simulink model "four_channel_bilateral_teleoperation_architecture"  (R2020b)
settings: Solver=VariableStepAuto  StartTime=0.0  StopTime=10.0  RelTol=1e-3
values from neighbouring files (symbols this model uses):
  A = 50    [four_channel_bilateral_teleoperation_architecture_params.m]    (also in four_channel_bilateral_teleoperation_kalman_params.m = 1; four_channel_bilateral_teleoperation_params.m = 1; kalman_test.m = [1 Ts Ts^2/2; 0 1 Ts; 0 0 1]; recursive_estimation.m = [1 Ts Ts^2/2; 0 1 Ts; 0 0 1])
  Be = 100    [four_channel_bilateral_teleoperation_architecture_params.m]    (also in four_channel_bilateral_teleoperation_kalman_params.m = 0; four_channel_bilateral_teleoperation_params.m = 0; scattering_based_bi_teleop_pf_kalman_params.m = 10; scattering_based_bi_teleop_pf_params.m = 10)
  Bh = 70    [four_channel_bilateral_teleoperation_architecture_params.m]    (also in four_channel_bilateral_teleoperation_kalman_params.m; four_channel_bilateral_teleoperation_params.m; scattering_based_bi_teleop_pf_kalman_params.m = 1.5; scattering_based_bi_teleop_pf_params.m = 1.5)
  Bm = 0.2    [four_channel_bilateral_teleoperation_architecture_params.m]    (also in four_channel_bilateral_teleoperation_kalman_params.m = 0.8; four_channel_bilateral_teleoperation_params.m = 0.8; scattering_based_bi_teleop_pf_kalman_params.m = 0; scattering_based_bi_teleop_pp_kalman_params.m = 15)
  Bs = 0.2    [four_channel_bilateral_teleoperation_architecture_params.m]    (also in four_channel_bilateral_teleoperation_kalman_params.m = 3.2; four_channel_bilateral_teleoperation_params.m = 3.2; scattering_based_bi_teleop_pf_kalman_params.m = 40; scattering_based_bi_teleop_pf_params.m = 3)
  Dh = 1.5    [four_channel_bilateral_teleoperation_architecture_params.m]    (also in four_channel_bilateral_teleoperation_kalman_params.m = 500; four_channel_bilateral_teleoperation_params.m = 100; scattering_based_bi_teleop_pf_kalman_params.m = 0; scattering_based_bi_teleop_pf_params.m = 17)
  Dm = 0    [four_channel_bilateral_teleoperation_architecture_params.m]    (also in four_channel_bilateral_teleoperation_kalman_params.m; four_channel_bilateral_teleoperation_params.m; scattering_based_bi_teleop_pf_kalman_params.m; scattering_based_bi_teleop_pf_params.m)
  Ds = 0    [four_channel_bilateral_teleoperation_architecture_params.m]    (also in four_channel_bilateral_teleoperation_kalman_params.m; four_channel_bilateral_teleoperation_params.m; scattering_based_bi_teleop_pf_kalman_params.m; scattering_based_bi_teleop_pf_params.m)
  Fc = 1    [four_channel_bilateral_teleoperation_architecture_params.m]    (also in four_channel_bilateral_teleoperation_kalman_params.m; four_channel_bilateral_teleoperation_params.m; kalman_test.m = 10; scattering_based_bi_teleop_pf_kalman_params.m = 0.1)
  Fip = 1    [four_channel_bilateral_teleoperation_architecture_params.m]    (also in four_channel_bilateral_teleoperation_kalman_params.m; four_channel_bilateral_teleoperation_params.m; scattering_based_bi_teleop_pf_kalman_params.m = 5; scattering_based_bi_teleop_pf_params.m)
  Je = 0    [four_channel_bilateral_teleoperation_architecture_params.m]    (also in four_channel_bilateral_teleoperation_kalman_params.m; four_channel_bilateral_teleoperation_params.m; scattering_based_bi_teleop_pf_kalman_params.m; scattering_based_bi_teleop_pf_params.m)
  Jh = 0.5    [four_channel_bilateral_teleoperation_architecture_params.m]    (also in four_channel_bilateral_teleoperation_kalman_params.m; four_channel_bilateral_teleoperation_params.m; scattering_based_bi_teleop_pf_kalman_params.m = 0; scattering_based_bi_teleop_pf_params.m = 0.05)
  Ke = 200    [four_channel_bilateral_teleoperation_architecture_params.m]    (also in four_channel_bilateral_teleoperation_kalman_params.m = 50; four_channel_bilateral_teleoperation_params.m; scattering_based_bi_teleop_pf_kalman_params.m; scattering_based_bi_teleop_pf_params.m)
  Kh = 2000    [four_channel_bilateral_teleoperation_architecture_params.m]    (also in four_channel_bilateral_teleoperation_kalman_params.m; four_channel_bilateral_teleoperation_params.m; scattering_based_bi_teleop_pf_kalman_params.m = 1; scattering_based_bi_teleop_pf_params.m = 0)
  Km = 30    [four_channel_bilateral_teleoperation_architecture_params.m]    (also in four_channel_bilateral_teleoperation_kalman_params.m = 1; four_channel_bilateral_teleoperation_params.m = 1; scattering_based_bi_teleop_pf_kalman_params.m = 0; scattering_based_bi_teleop_pp_kalman_params.m = 10)
  Ks = 30    [four_channel_bilateral_teleoperation_architecture_params.m]    (also in four_channel_bilateral_teleoperation_kalman_params.m = 4; four_channel_bilateral_teleoperation_params.m = 4; scattering_based_bi_teleop_pf_kalman_params.m = 50; scattering_based_bi_teleop_pf_params.m = 110)
  Mm = 0.5    [four_channel_bilateral_teleoperation_architecture_params.m]    (also in four_channel_bilateral_teleoperation_kalman_params.m; four_channel_bilateral_teleoperation_params.m; scattering_based_bi_teleop_pf_kalman_params.m; scattering_based_bi_teleop_pf_params.m)
  Ms = 2    [four_channel_bilateral_teleoperation_architecture_params.m]    (also in four_channel_bilateral_teleoperation_kalman_params.m; four_channel_bilateral_teleoperation_params.m; scattering_based_bi_teleop_pf_kalman_params.m; scattering_based_bi_teleop_pf_params.m)
  Ph = 0.2    [four_channel_bilateral_teleoperation_architecture_params.m]    (also in four_channel_bilateral_teleoperation_kalman_params.m = 2000; four_channel_bilateral_teleoperation_params.m = 20100; scattering_based_bi_teleop_pf_kalman_params.m = 5; scattering_based_bi_teleop_pf_params.m = 23)
  tau = 10000    [four_channel_bilateral_teleoperation_architecture_params.m]
settings Model: Creator=anuj  LastModifiedBy=filippo

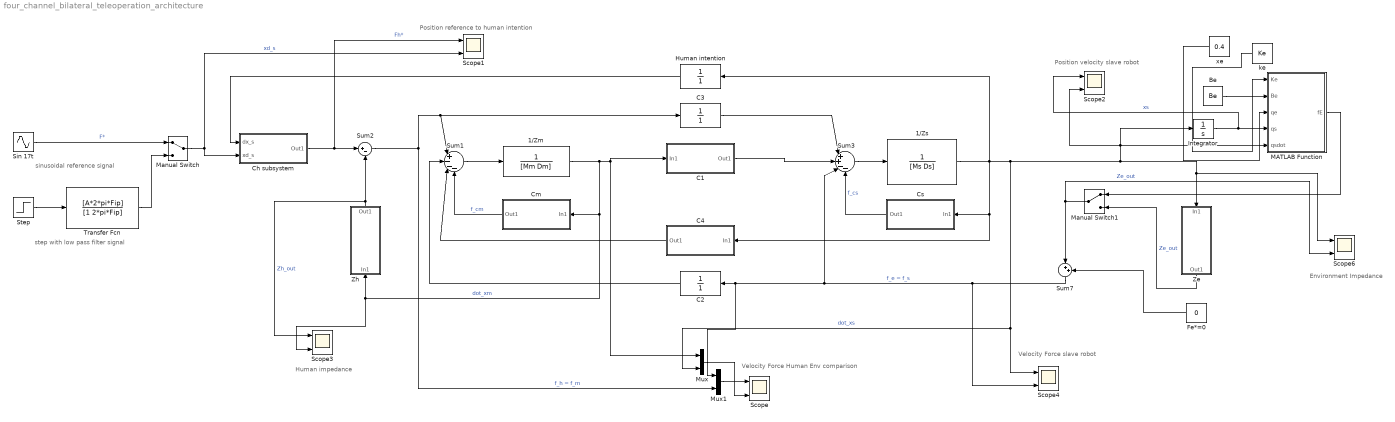
== system four_channel_bilateral_teleoperation_architecture ==
  note: Environment Impedance
  note: Human impedance
  note: Velocity Force Human Env comparison
  note: Velocity Force slave robot
  note: Position velocity slave robot
  note: sinusoidal reference signal
  note: step with low pass filter signal
  note: Position reference to human intention
  1/Zm : TransferFcn  Denominator=[Mm Dm]
  1/Zs : TransferFcn  Denominator=[Ms Ds]
  Be : Constant  Value=Be
  C1 : Subsystem
  C2 : TransferFcn  Denominator=[1]
  C3 : TransferFcn  Denominator=[1]
  C4 : Subsystem
  Ch subsystem : Subsystem
  Cm : Subsystem
  Cs : Subsystem
  Fe*=0 : Constant  Value=0
  Human intention : TransferFcn  Denominator=[1]
  Integrator : Integrator
  MATLAB Function : MATLAB Function  TreatAsAtomicUnit=on
  Manual Switch : ManualSwitch
  Manual Switch1 : ManualSwitch
  Mux : Mux  Inputs=2
  Mux1 : Mux  Inputs=2
  Scope{,1..4,6} (6 alike) : Scope  NumInputPorts=2
  Sin 17t : Sin  Amplitude=A  Frequency=2*pi*Fc  SampleTime=0
  Step : Step  SampleTime=0
  Sum1 : Sum  Inputs=|+---
  Sum2 : Sum  Inputs=|+-
  Sum3 : Sum  Inputs=|++--
  Sum7 : Sum  Inputs=|++
  Transfer Fcn : TransferFcn  Numerator=[A*2*pi*Fip]  Denominator=[1 2*pi*Fip]
  Ze : Subsystem
  Zh : Subsystem
  ke : Constant  Value=Ke
  xe : Constant  Value=0.4
  wires:
  Mux/1 -> Scope/2
  Mux1/1 -> Scope/1
  Sum2/1 -> Sum1/1, C3/1, Mux1/2  "f_h = f_m"
  1/Zm/1 -> C1/1(In1), Mux/1, Zh/1(In1), Scope3/2, Cm/1(In1)  "dot_xm"
  Sum1/1 -> 1/Zm/1
  C2/1 -> Sum1/2
  C3/1 -> Sum3/1
  Sum3/1 -> 1/Zs/1
  Fe*=0/1 -> Sum7/2
  Sum7/1 -> Sum3/3, Mux1/1, C2/1, Scope4/2  "f_e = f_s"
  C4/1(Out1) -> Sum1/3
  Ch subsystem/1(Out1) -> Scope1/1, Sum2/1  "Fh*"
  Be/1 -> MATLAB Function/2(Be)
  xe/1 -> MATLAB Function/3(qe)
  ke/1 -> MATLAB Function/1(Ke)
  Integrator/1 -> Scope2/1, MATLAB Function/4(qs)  "xs"
  Transfer Fcn/1 -> Manual Switch/2
  Step/1 -> Transfer Fcn/1
  Human intention/1 -> Ch subsystem/1(dx_s)
  Manual Switch/1 -> Ch subsystem/2(xd_s), Scope1/2  "xd_s"
  Sin 17t/1 -> Manual Switch/1  "F*"
  C1/1(Out1) -> Sum3/2
  MATLAB Function/1(fE) -> Manual Switch1/1
  1/Zs/1 -> C4/1(In1), Cs/1(In1), Scope4/1, Mux/2, MATLAB Function/5(qsdot), Scope2/2, Integrator/1, Scope6/1, Ze/1(In1), Human intention/1  "dot_xs"
  Manual Switch1/1 -> Sum7/1, Scope6/2  "Ze_out"
  Zh/1(Out1) -> Sum2/2, Scope3/1  "Zh_out"
  Cm/1(Out1) -> Sum1/4  "f_cm"
  Cs/1(Out1) -> Sum3/4  "f_cs"
  Ze/1(Out1) -> Manual Switch1/2  "Ze_out"

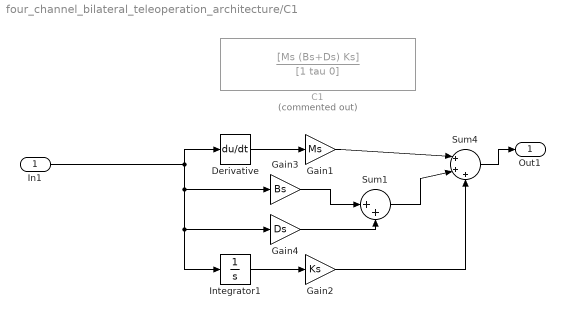
== system four_channel_bilateral_teleoperation_architecture/C1 ==
  In1 : Inport
  C1 : TransferFcn  Commented=on  Numerator=[Ms (Bs+Ds) Ks]  Denominator=[1 tau 0]
  Derivative : Derivative
  Gain1 : Gain  Gain=Ms
  Gain2 : Gain  Gain=Ks
  Gain3 : Gain  Gain=Bs
  Gain4 : Gain  Gain=Ds
  Integrator1 : Integrator
  Sum1 : Sum  Inputs=|++
  Sum4 : Sum  Inputs=|+++
  Out1 : Outport
  wires:
  Sum4/1 -> Out1/1
  Gain1/1 -> Sum4/1
  Integrator1/1 -> Gain2/1
  In1/1 -> Derivative/1, Gain3/1, Integrator1/1, Gain4/1
  Gain2/1 -> Sum4/3
  Sum1/1 -> Sum4/2
  Gain4/1 -> Sum1/2
  Gain3/1 -> Sum1/1
  Derivative/1 -> Gain1/1

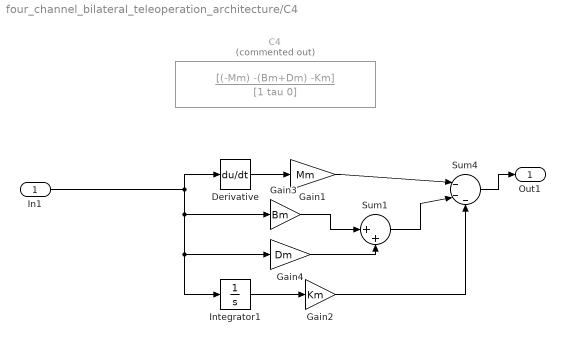
== system four_channel_bilateral_teleoperation_architecture/C4 ==
  In1 : Inport
  C4 : TransferFcn  Commented=on  Numerator=[(-Mm) -(Bm+Dm) -Km]  Denominator=[1 tau 0]
  Derivative : Derivative
  Gain1 : Gain  Gain=Mm
  Gain2 : Gain  Gain=Km
  Gain3 : Gain  Gain=Bm
  Gain4 : Gain  Gain=Dm
  Integrator1 : Integrator
  Sum1 : Sum  Inputs=|++
  Sum4 : Sum  Inputs=|---
  Out1 : Outport
  wires:
  Sum4/1 -> Out1/1
  Gain1/1 -> Sum4/1
  Integrator1/1 -> Gain2/1
  In1/1 -> Derivative/1, Gain3/1, Integrator1/1, Gain4/1
  Gain2/1 -> Sum4/3
  Sum1/1 -> Sum4/2
  Gain4/1 -> Sum1/2
  Gain3/1 -> Sum1/1
  Derivative/1 -> Gain1/1

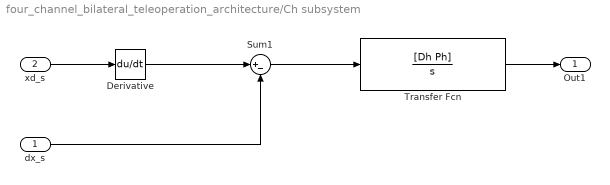
== system four_channel_bilateral_teleoperation_architecture/Ch subsystem ==
  dx_s : Inport
  xd_s : Inport  Port=2
  Derivative : Derivative
  Sum1 : Sum  Inputs=|+-
  Transfer Fcn : TransferFcn  Numerator=[Dh Ph]  Denominator=[1 0]
  Out1 : Outport
  wires:
  dx_s/1 -> Sum1/2
  Sum1/1 -> Transfer Fcn/1
  xd_s/1 -> Derivative/1
  Derivative/1 -> Sum1/1
  Transfer Fcn/1 -> Out1/1

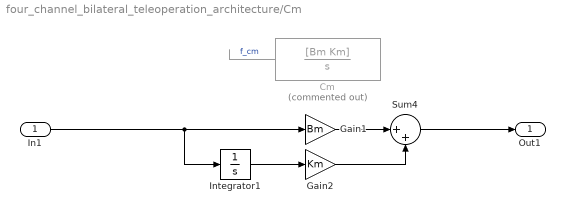
== system four_channel_bilateral_teleoperation_architecture/Cm ==
  In1 : Inport
  Cm : TransferFcn  Commented=on  Numerator=[Bm Km]  Denominator=[1 0]
  Gain1 : Gain  Gain=Bm
  Gain2 : Gain  Gain=Km
  Integrator1 : Integrator
  Sum4 : Sum  Inputs=|++
  Out1 : Outport
  wires:
  Sum4/1 -> Out1/1
  Gain1/1 -> Sum4/1
  Integrator1/1 -> Gain2/1
  In1/1 -> Gain1/1, Integrator1/1
  Gain2/1 -> Sum4/2
  Cm/1 -> ?  "f_cm"

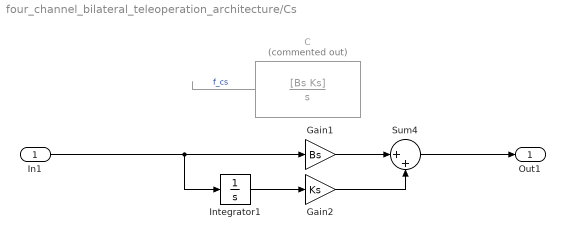
== system four_channel_bilateral_teleoperation_architecture/Cs ==
  In1 : Inport
  C : TransferFcn  Commented=on  Numerator=[Bs Ks]  Denominator=[1 0]
  Gain1 : Gain  Gain=Bs
  Gain2 : Gain  Gain=Ks
  Integrator1 : Integrator
  Sum4 : Sum  Inputs=|++
  Out1 : Outport
  wires:
  Sum4/1 -> Out1/1
  Gain1/1 -> Sum4/1
  Integrator1/1 -> Gain2/1
  In1/1 -> Gain1/1, Integrator1/1
  Gain2/1 -> Sum4/2
  C/1 -> ?  "f_cs"

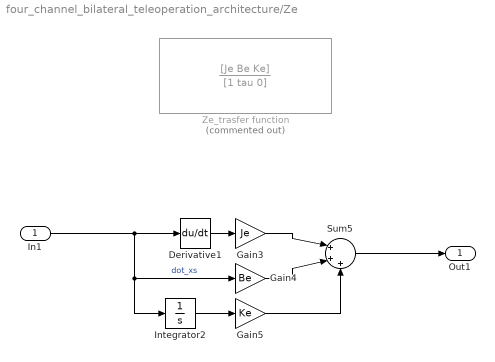
== system four_channel_bilateral_teleoperation_architecture/Ze ==
  In1 : Inport
  Derivative1 : Derivative
  Gain3 : Gain  Gain=Je
  Gain4 : Gain  Gain=Be
  Gain5 : Gain  Gain=Ke
  Integrator2 : Integrator
  Sum5 : Sum  Inputs=|+++
  Ze_trasfer function : TransferFcn  Commented=on  Numerator=[Je Be Ke]  Denominator=[1 tau 0]
  Out1 : Outport
  wires:
  Gain4/1 -> Sum5/2
  Gain3/1 -> Sum5/1
  Gain5/1 -> Sum5/3
  Sum5/1 -> Out1/1
  Integrator2/1 -> Gain5/1
  In1/1 -> Integrator2/1, Gain4/1, Derivative1/1  "dot_xs"
  Derivative1/1 -> Gain3/1

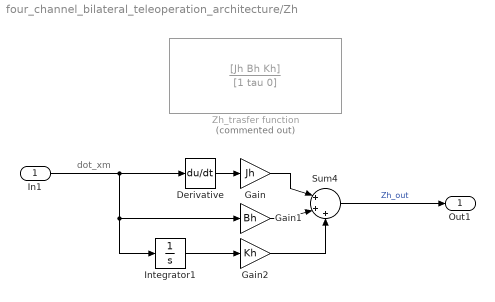
== system four_channel_bilateral_teleoperation_architecture/Zh ==
  note: dot_xm
  In1 : Inport
  Derivative : Derivative
  Gain : Gain  Gain=Jh
  Gain1 : Gain  Gain=Bh
  Gain2 : Gain  Gain=Kh
  Integrator1 : Integrator
  Sum4 : Sum  Inputs=|+++
  Zh_trasfer function : TransferFcn  Commented=on  Numerator=[Jh Bh Kh]  Denominator=[1 tau 0]
  Out1 : Outport
  wires:
  Derivative/1 -> Gain/1
  Integrator1/1 -> Gain2/1
  Gain2/1 -> Sum4/3
  Gain1/1 -> Sum4/2
  Gain/1 -> Sum4/1
  Sum4/1 -> Out1/1  "Zh_out"
  In1/1 -> Gain1/1, Integrator1/1, Derivative/1

== matlab function four_channel_bilateral_teleoperation_architecture/MATLAB Function ==
  data: Ke input; fE output; Be input; qe input; qs input; qsdot input
function fE = environment(Ke, Be, qe, qs, qsdot)
    if qs > qe
        fE = Ke * (qs - qe) + Be * qsdot;
    else
        fE = 0;
    end
end
